simulink model "BESSmodel_EMT"  (R2019a)
settings: Solver=FixedStepAuto  SolverName=VariableStepAuto  StartTime=0.0  StopTime=10  RelTol=1e-3
undefined symbols (not defined in the file): D11, Delta, Ion, Lithium
libraries: powerlib x24, powerlib_meascontrol x15, simulink x9, eeGeneralControl x8, electricdrivelib x1
(part 2 of 2)

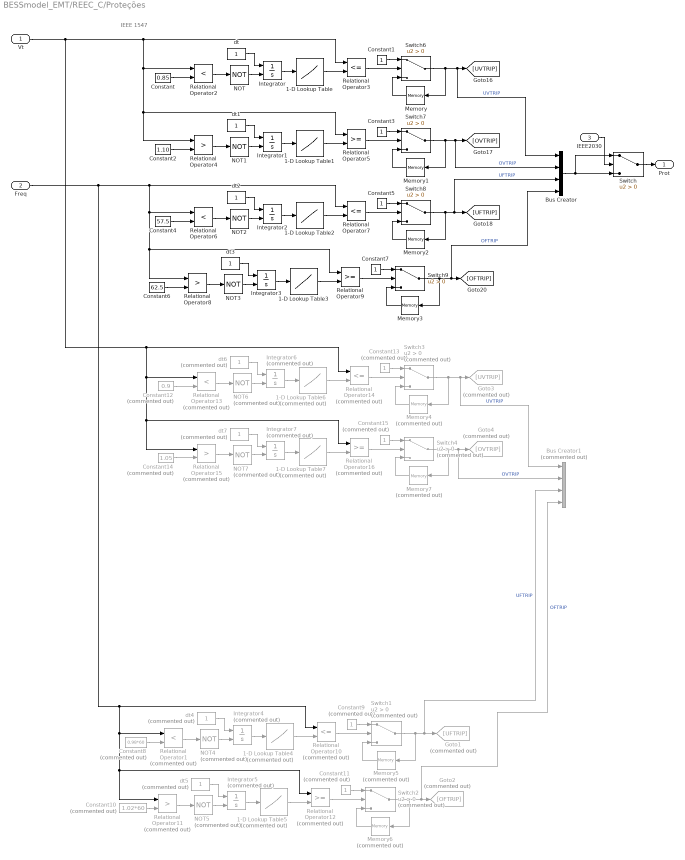
== system BESSmodel_EMT/REEC_C/Proteções ==
  note: IEEE 1547
  Vt : Inport
  Freq : Inport  Port=2
  IEEE2030 : Inport  Port=3
  1-D Lookup Table : Lookup_n-D  NumberOfTableDimensions=1  BreakpointsForDimension1=[0;0.31;0.3101;4;4.0001;99999]  Table=[0.0001;0.15;0.1501;0.15;0.8501;0.85]  InternalRulePriority=Speed  RndMeth=Simplest  InputSameDT=on
  1-D Lookup Table1 : Lookup_n-D  NumberOfTableDimensions=1  BreakpointsForDimension1=[0;0.3;0.3001;2.1;2.1001;99999]  Table=[99999.0001;1.2;1.2001;1.2;1.1001;1.1]  InternalRulePriority=Speed  RndMeth=Simplest  InputSameDT=on
  1-D Lookup Table2 : Lookup_n-D  NumberOfTableDimensions=1  BreakpointsForDimension1=[0;0.08;0.0801;10;10.0001;99999]  Table=[50.0001;57.499;57.4991;57.499;57.5001;57.5]  InternalRulePriority=Speed  RndMeth=Simplest  InputSameDT=on
  1-D Lookup Table3 : Lookup_n-D  NumberOfTableDimensions=1  BreakpointsForDimension1=[0;0.08;0.0801;10;10.0001;99999]  Table=[70.0001;62.499;62.4991;62.499;62.5001;62.5]  InternalRulePriority=Speed  RndMeth=Simplest  InputSameDT=on
  1-D Lookup Table4 : Lookup_n-D  Commented=on  NumberOfTableDimensions=1  BreakpointsForDimension1=[0;299;299.0001;100000]  Table=[57;57;58.8;58.8]  InternalRulePriority=Speed  RndMeth=Simplest  InputSameDT=on
  1-D Lookup Table5 : Lookup_n-D  Commented=on  NumberOfTableDimensions=1  BreakpointsForDimension1=[0;299;299.0001;100000]  Table=[61.8;61.8;61.2;61.2]  InternalRulePriority=Speed  RndMeth=Simplest  InputSameDT=on
  1-D Lookup Table6 : Lookup_n-D  Commented=on  NumberOfTableDimensions=1  BreakpointsForDimension1=[0;0.31;0.3101;4;4.0001;99999]  Table=[0.0001;0.15;0.1501;0.15;0.8501;0.85]  InternalRulePriority=Speed  RndMeth=Simplest  InputSameDT=on
  1-D Lookup Table7 : Lookup_n-D  Commented=on  NumberOfTableDimensions=1  BreakpointsForDimension1=[0;0.3;0.3001;2.1;2.1001;99999]  Table=[99999.0001;1.2;1.2001;1.2;1.1001;1.1]  InternalRulePriority=Speed  RndMeth=Simplest  InputSameDT=on
  Bus Creator : BusCreator  Inputs=4
  Bus Creator1 : BusCreator  Commented=on  Inputs=4
  Constant : Constant  Value=0.85
  Constant{1,3,5,7} (4 alike) : Constant
  Constant10 : Constant  Commented=on  Value=1.02*60
  Constant{9,11,13,15} (4 alike) : Constant  Commented=on
  Constant12 : Constant  Commented=on  Value=0.9
  Constant14 : Constant  Commented=on  Value=1.05
  Constant2 : Constant  Value=1.10
  Constant4 : Constant  Value=57.5
  Constant6 : Constant  Value=62.5
  Constant8 : Constant  Commented=on  Value=0.98*60
  Goto1 : Goto  Commented=on  GotoTag=UFTRIP
  Goto2 : Goto  Commented=on  GotoTag=OFTRIP
  Goto3 : Goto  Commented=on  GotoTag=UVTRIP
  Goto4 : Goto  Commented=on  GotoTag=OVTRIP
  Integrator{,1..3} (4 alike) : Integrator  ExternalReset=level
  Integrator4 : Integrator  Commented=on  ExternalReset=level
  Integrator5 : Integrator  Commented=on  ExternalReset=level
  Integrator6 : Integrator  Commented=on  ExternalReset=level
  Integrator7 : Integrator  Commented=on  ExternalReset=level hold
  Memory{,1..3} (4 alike) : Memory
  Memory{4..7} (4 alike) : Memory  Commented=on
  NOT{,1..3} (4 alike) : Logic  Operator=NOT  IconShape=distinctive  AllPortsSameDT=off  OutDataTypeStr=boolean
  NOT{4..7} (4 alike) : Logic  Commented=on  Operator=NOT  IconShape=distinctive  AllPortsSameDT=off  OutDataTypeStr=boolean
  Relational Operator1 : RelationalOperator  Commented=on  Operator=<  OutDataTypeStr=boolean  RndMeth=Simplest
  Relational Operator10 : RelationalOperator  Commented=on  Operator=<=  OutDataTypeStr=boolean  RndMeth=Simplest
  Relational Operator11 : RelationalOperator  Commented=on  Operator=>  OutDataTypeStr=boolean  RndMeth=Simplest
  Relational Operator12 : RelationalOperator  Commented=on  OutDataTypeStr=boolean  RndMeth=Simplest
  Relational Operator13 : RelationalOperator  Commented=on  Operator=<  OutDataTypeStr=boolean  RndMeth=Simplest
  Relational Operator14 : RelationalOperator  Commented=on  Operator=<=  OutDataTypeStr=boolean  RndMeth=Simplest
  Relational Operator15 : RelationalOperator  Commented=on  Operator=>  OutDataTypeStr=boolean  RndMeth=Simplest
  Relational Operator16 : RelationalOperator  Commented=on  OutDataTypeStr=boolean  RndMeth=Simplest
  Relational Operator2 : RelationalOperator  Operator=<  OutDataTypeStr=boolean  RndMeth=Simplest
  Relational Operator3 : RelationalOperator  Operator=<=  OutDataTypeStr=boolean  RndMeth=Simplest
  Relational Operator4 : RelationalOperator  Operator=>  OutDataTypeStr=boolean  RndMeth=Simplest
  Relational Operator5 : RelationalOperator  OutDataTypeStr=boolean  RndMeth=Simplest
  Relational Operator6 : RelationalOperator  Operator=<  OutDataTypeStr=boolean  RndMeth=Simplest
  Relational Operator7 : RelationalOperator  Operator=<=  OutDataTypeStr=boolean  RndMeth=Simplest
  Relational Operator8 : RelationalOperator  Operator=>  OutDataTypeStr=boolean  RndMeth=Simplest
  Relational Operator9 : RelationalOperator  OutDataTypeStr=boolean  RndMeth=Simplest
  Switch{,6..9} (5 alike) : Switch  Criteria=u2 > Threshold
  Switch{1..4} (4 alike) : Switch  Commented=on  Criteria=u2 > Threshold
  dt{,1..3} (4 alike) : Constant
  dt{4..7} (4 alike) : Constant  Commented=on
  Prot : Outport
  wires:
  Integrator/1 -> 1-D Lookup Table/1
  Constant5/1 -> Switch8/1
  Switch8/1 -> Bus Creator/3, [UFTRIP], Memory2/1  "UFTRIP"
  Switch7/1 -> Bus Creator/2, [OVTRIP], Memory1/1  "OVTRIP"
  Memory2/1 -> Switch8/3
  Integrator1/1 -> 1-D Lookup Table1/1
  Relational Operator3/1 -> Switch6/2
  Relational Operator2/1 -> NOT/1
  Switch6/1 -> Bus Creator/1, [UVTRIP], Memory/1  "UVTRIP"
  NOT/1 -> Integrator/2
  dt/1 -> Integrator/1
  Relational Operator8/1 -> NOT3/1
  1-D Lookup Table/1 -> Relational Operator3/2
  Constant/1 -> Relational Operator2/2
  Integrator3/1 -> 1-D Lookup Table3/1
  Switch9/1 -> Bus Creator/4, [OFTRIP], Memory3/1  "OFTRIP"
  Relational Operator5/1 -> Switch7/2
  Relational Operator9/1 -> Switch9/2
  1-D Lookup Table1/1 -> Relational Operator5/2
  dt1/1 -> Integrator1/1
  Memory/1 -> Switch6/3
  Constant4/1 -> Relational Operator6/2
  Constant1/1 -> Switch6/1
  dt3/1 -> Integrator3/1
  Constant7/1 -> Switch9/1
  dt2/1 -> Integrator2/1
  NOT1/1 -> Integrator1/2
  Constant2/1 -> Relational Operator4/2
  NOT2/1 -> Integrator2/2
  Relational Operator6/1 -> NOT2/1
  Relational Operator7/1 -> Switch8/2
  Integrator2/1 -> 1-D Lookup Table2/1
  1-D Lookup Table3/1 -> Relational Operator9/2
  NOT3/1 -> Integrator3/2
  Memory3/1 -> Switch9/3
  Memory1/1 -> Switch7/3
  Relational Operator4/1 -> NOT1/1
  Constant3/1 -> Switch7/1
  1-D Lookup Table2/1 -> Relational Operator7/2
  Constant6/1 -> Relational Operator8/2
  Bus Creator/1 -> Switch/1, Switch/3
  Switch/1 -> Prot/1
  IEEE2030/1 -> Switch/2
  Relational Operator1/1 -> NOT4/1
  Relational Operator11/1 -> NOT5/1
  1-D Lookup Table4/1 -> Relational Operator10/2
  NOT4/1 -> Integrator4/2
  Constant10/1 -> Relational Operator11/2
  1-D Lookup Table5/1 -> Relational Operator12/2
  dt4/1 -> Integrator4/1
  Constant11/1 -> Switch2/1
  NOT5/1 -> Integrator5/2
  Integrator4/1 -> 1-D Lookup Table4/1
  Constant8/1 -> Relational Operator1/2
  Relational Operator12/1 -> Switch2/2
  Relational Operator10/1 -> Switch1/2
  Switch1/1 -> Bus Creator1/3, Goto1/1, Memory5/1  "UFTRIP"
  Integrator5/1 -> 1-D Lookup Table5/1
  dt5/1 -> Integrator5/1
  Constant9/1 -> Switch1/1
  Switch2/1 -> Bus Creator1/4, Goto2/1, Memory6/1  "OFTRIP"
  Memory5/1 -> Switch1/3
  Memory6/1 -> Switch2/3
  Freq/1 -> Relational Operator1/1, Relational Operator12/1, Relational Operator11/1, Relational Operator10/1, Relational Operator6/1, Relational Operator9/1, Relational Operator8/1, Relational Operator7/1
  Constant13/1 -> Switch3/1
  Vt/1 -> Relational Operator14/1, Relational Operator13/1, Relational Operator16/1, Relational Operator15/1, Relational Operator3/1, Relational Operator2/1, Relational Operator5/1, Relational Operator4/1
  Relational Operator15/1 -> NOT7/1
  Integrator6/1 -> 1-D Lookup Table6/1
  NOT6/1 -> Integrator6/2
  Memory7/1 -> Switch4/3
  Constant14/1 -> Relational Operator15/2
  Constant15/1 -> Switch4/1
  NOT7/1 -> Integrator7/2
  1-D Lookup Table7/1 -> Relational Operator16/2
  Memory4/1 -> Switch3/3
  Relational Operator16/1 -> Switch4/2
  dt6/1 -> Integrator6/1
  dt7/1 -> Integrator7/1
  1-D Lookup Table6/1 -> Relational Operator14/2
  Integrator7/1 -> 1-D Lookup Table7/1
  Switch3/1 -> Bus Creator1/1, Goto3/1, Memory4/1  "UVTRIP"
  Constant12/1 -> Relational Operator13/2
  Relational Operator13/1 -> NOT6/1
  Relational Operator14/1 -> Switch3/2
  Switch4/1 -> Bus Creator1/2, Goto4/1, Memory7/1  "OVTRIP"

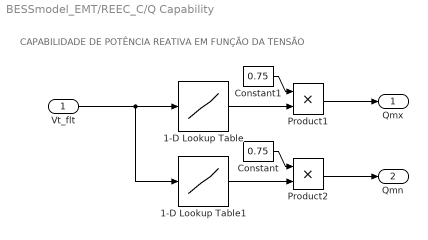
== system BESSmodel_EMT/REEC_C/Q Capability ==
  note: CAPABILIDADE DE POTÊNCIA REATIVA EM FUNÇÃO DA TENSÃO
  Vt_flt : Inport
  1-D Lookup Table : Lookup_n-D  NumberOfTableDimensions=1  BreakpointsForDimension1=[0.9;0.95;1.03;1.05]  Table=[0.7;1;1;0]  InternalRulePriority=Speed  RndMeth=Simplest  InputSameDT=on
  1-D Lookup Table1 : Lookup_n-D  NumberOfTableDimensions=1  BreakpointsForDimension1=[0.95;0.99;1.05;1.0501]  Table=[0;-1;-1;0]  InternalRulePriority=Speed  RndMeth=Simplest  InputSameDT=on
  Constant : Constant  Value=0.75
  Constant1 : Constant  Value=0.75
  Product1 : Product
  Product2 : Product
  Qmx : Outport
  Qmn : Outport  Port=2
  wires:
  Constant1/1 -> Product1/1
  1-D Lookup Table/1 -> Product1/2
  1-D Lookup Table1/1 -> Product2/2
  Vt_flt/1 -> 1-D Lookup Table1/1, 1-D Lookup Table/1
  Constant/1 -> Product2/1
  Product2/1 -> Qmn/1
  Product1/1 -> Qmx/1

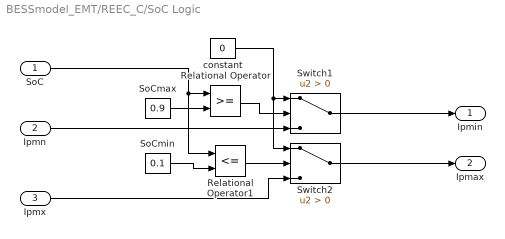
== system BESSmodel_EMT/REEC_C/SoC Logic ==
  SoC : Inport
  Ipmn : Inport  Port=2
  Ipmx : Inport  Port=3
  Relational Operator : RelationalOperator  OutDataTypeStr=boolean  RndMeth=Simplest
  Relational Operator1 : RelationalOperator  Operator=<=  OutDataTypeStr=boolean  RndMeth=Simplest
  SoCmax : Constant  Value=0.9
  SoCmin : Constant  Value=0.1
  Switch1 : Switch  Criteria=u2 > Threshold
  Switch2 : Switch  Criteria=u2 > Threshold
  constant : Constant  Value=0
  Ipmin : Outport
  Ipmax : Outport  Port=2
  wires:
  SoC/1 -> Relational Operator/1, Relational Operator1/1
  Ipmx/1 -> Switch2/3
  constant/1 -> Switch2/1, Switch1/1
  Switch1/1 -> Ipmin/1
  Relational Operator1/1 -> Switch2/2
  Relational Operator/1 -> Switch1/2
  SoCmax/1 -> Relational Operator/2
  SoCmin/1 -> Relational Operator1/2
  Ipmn/1 -> Switch1/3
  Switch2/1 -> Ipmax/1

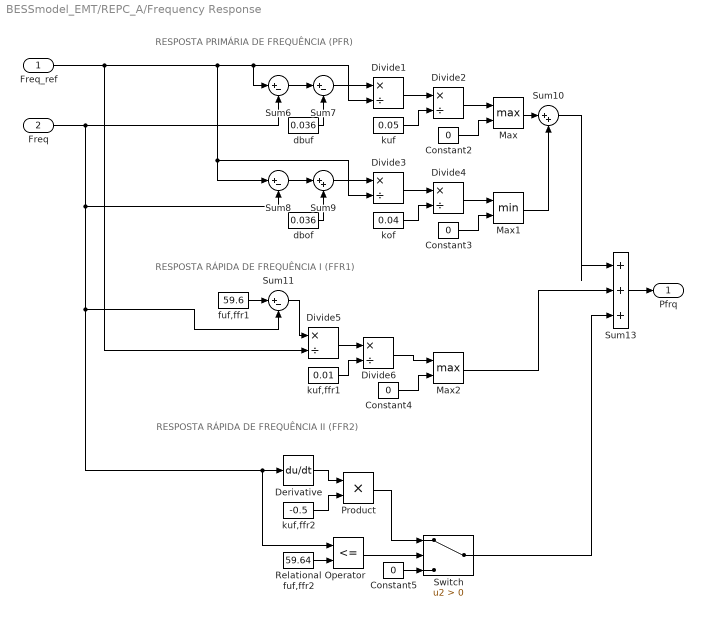
== system BESSmodel_EMT/REPC_A/Frequency Response ==
  note: RESPOSTA RÁPIDA DE FREQUÊNCIA II (FFR2)
  note: RESPOSTA RÁPIDA DE FREQUÊNCIA I (FFR1)
  note: RESPOSTA PRIMÁRIA DE FREQUÊNCIA (PFR)
  Freq_ref : Inport
  Freq : Inport  Port=2
  Constant{2..5} (4 alike) : Constant  Value=0
  Derivative : Derivative
  Divide{1..6} (6 alike) : Product  Inputs=*/
  Max : MinMax  Function=max  Inputs=2
  Max1 : MinMax  Inputs=2
  Max2 : MinMax  Function=max  Inputs=2
  Product : Product
  Relational Operator : RelationalOperator  Operator=<=  OutDataTypeStr=boolean  RndMeth=Simplest
  Sum10 : Sum  Inputs=|++
  Sum{6..8,11} (4 alike) : Sum  Inputs=|+-
  Sum13 : Sum  Inputs=|+++
  Sum9 : Sum  Inputs=|++
  Switch : Switch  Criteria=u2 > Threshold
  dbof : Constant  Value=0.036
  dbuf : Constant  Value=0.036
  fuf,ffr1 : Constant  Value=59.6
  fuf,ffr2 : Constant  Value=59.64
  kof : Constant  Value=0.04
  kuf : Constant  Value=0.05
  kuf,ffr1 : Constant  Value=0.01
  kuf,ffr2 : Constant  Value=-0.5
  Pfrq : Outport
  wires:
  Sum10/1 -> Sum13/1
  Max/1 -> Sum10/1
  Freq/1 -> Sum6/2, Sum8/2, Sum11/2, Relational Operator/1, Derivative/1
  Freq_ref/1 -> Divide3/2, Sum8/1, Sum6/1, Divide1/2, Divide5/2
  Sum11/1 -> Divide5/1
  Sum9/1 -> Divide3/1
  Sum8/1 -> Sum9/1
  kuf,ffr2/1 -> Product/2
  Divide5/1 -> Divide6/1
  kuf/1 -> Divide2/2
  Constant3/1 -> Max1/2
  dbuf/1 -> Sum7/2
  dbof/1 -> Sum9/2
  kof/1 -> Divide4/2
  Divide4/1 -> Max1/1
  Max2/1 -> Sum13/2
  Derivative/1 -> Product/1
  Constant5/1 -> Switch/3
  Divide1/1 -> Divide2/1
  Product/1 -> Switch/1
  Divide2/1 -> Max/1
  fuf,ffr1/1 -> Sum11/1
  Sum13/1 -> Pfrq/1
  kuf,ffr1/1 -> Divide6/2
  Sum7/1 -> Divide1/1
  Constant2/1 -> Max/2
  Constant4/1 -> Max2/2
  Divide3/1 -> Divide4/1
  Sum6/1 -> Sum7/1
  Switch/1 -> Sum13/3
  Max1/1 -> Sum10/2
  fuf,ffr2/1 -> Relational Operator/2
  Relational Operator/1 -> Switch/2
  Divide6/1 -> Max2/1

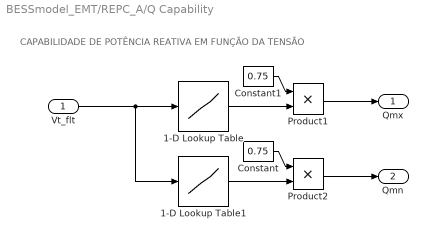
== system BESSmodel_EMT/REPC_A/Q Capability ==
  note: CAPABILIDADE DE POTÊNCIA REATIVA EM FUNÇÃO DA TENSÃO
  Vt_flt : Inport
  1-D Lookup Table : Lookup_n-D  NumberOfTableDimensions=1  BreakpointsForDimension1=[0.9;0.95;1.03;1.05]  Table=[0.7;1;1;0]  InternalRulePriority=Speed  RndMeth=Simplest  InputSameDT=on
  1-D Lookup Table1 : Lookup_n-D  NumberOfTableDimensions=1  BreakpointsForDimension1=[0.95;0.99;1.05;1.0501]  Table=[0;-1;-1;0]  InternalRulePriority=Speed  RndMeth=Simplest  InputSameDT=on
  Constant : Constant  Value=0.75
  Constant1 : Constant  Value=0.75
  Product1 : Product
  Product2 : Product
  Qmx : Outport
  Qmn : Outport  Port=2
  wires:
  Constant1/1 -> Product1/1
  1-D Lookup Table/1 -> Product1/2
  1-D Lookup Table1/1 -> Product2/2
  Vt_flt/1 -> 1-D Lookup Table1/1, 1-D Lookup Table/1
  Constant/1 -> Product2/1
  Product2/1 -> Qmn/1
  Product1/1 -> Qmx/1
